simulink model "ClassExampleMar24"  (R2018b)
settings: Solver=VariableStepAuto  StartTime=0.0  StopTime=4  RelTol=1e-3
settings Model: Creator=diduch  LastModifiedBy=diduch

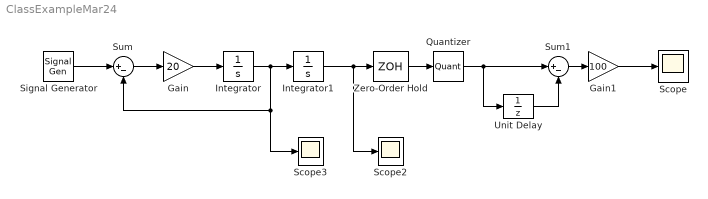
== system ClassExampleMar24 ==
  Gain : Gain  Gain=20
  Gain1 : Gain  Gain=100
  Integrator : Integrator
  Integrator1 : Integrator
  Quantizer : Quantizer  QuantizationInterval=2*pi/16
  Scope : Scope
  Scope2 : Scope
  Scope3 : Scope
  Signal Generator : SignalGenerator  WaveForm=square  Amplitude=1000  Frequency=.5
  Sum : Sum  Inputs=|+-
  Sum1 : Sum  Inputs=|+-
  Unit Delay : UnitDelay  SampleTime=-1
  Zero-Order Hold : ZeroOrderHold  SampleTime=0.01
  wires:
  Integrator/1 -> Integrator1/1, Scope3/1, Sum/2
  Gain/1 -> Integrator/1
  Sum/1 -> Gain/1
  Integrator1/1 -> Scope2/1, Zero-Order Hold/1
  Zero-Order Hold/1 -> Quantizer/1
  Quantizer/1 -> Sum1/1, Unit Delay/1
  Unit Delay/1 -> Sum1/2
  Sum1/1 -> Gain1/1
  Gain1/1 -> Scope/1
  Signal Generator/1 -> Sum/1
